simulink model "pha_0_5_servovalve"  (R2023a)
settings: Solver=VariableStepAuto  StartTime=0.0  StopTime=15  RelTol=1e-3
libraries: fl_lib x82, SimscapeFluids_lib x26, nesl_utility x8
(part 1 of 2)
Description:
  | Model contains pump, accumulator, relief valve for pump and accumulator
  | as well as 3-way directional valves. The point of this example is to show how
  | the pressure in accumulator chamber can be controlled to be between 1.4 and 1.5 bars
settings Model: Creator=Dovlica  LastModifiedBy=Dovlica
settings SimscapeCC: SimscapeLogType=all

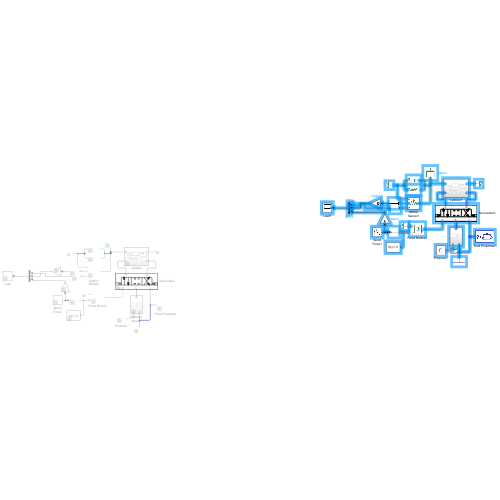
[thumbnail: Simulink's stored preview of the top-level diagram]
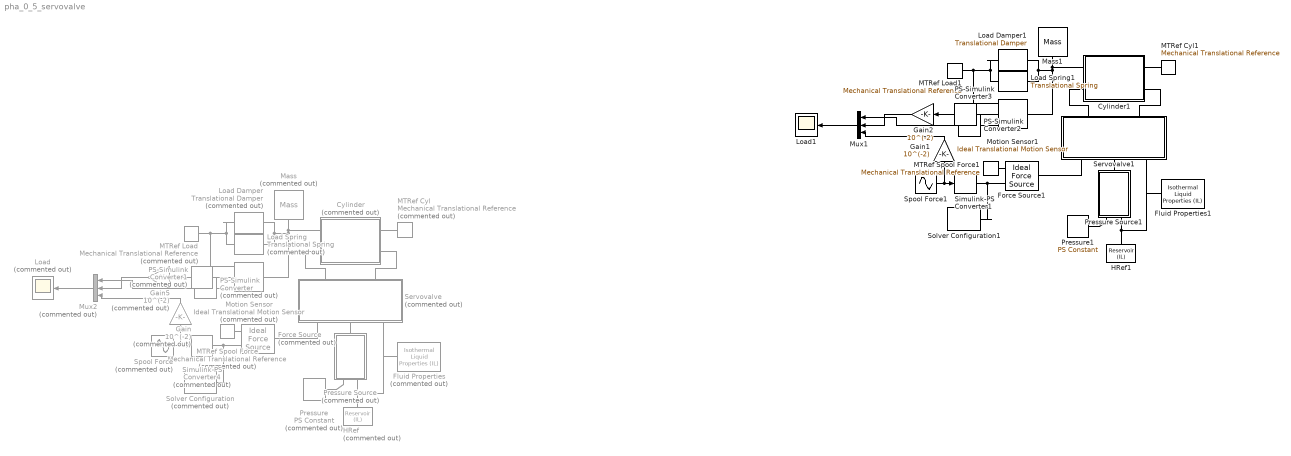
== system pha_0_5_servovalve ==
  " Fluid Properties" : fl_lib/Isothermal Liquid/Utilities/Isothermal Liquid Properties (IL)  Tag=Factory Generic  Commented=on  rho_L_atm=832.816 kg/m^3  bulk_modulus_model=foundation.enum.bulk_modulus_model.const  beta_gain=6  beta_L_atm=1.56078e+09 Pa  nu_atm=(3.9468)*(1) cSt  p_atm=0.101325 MPa  p_min=1 Pa  properties_range_check=simscape.enum.assert.action.error  air_fraction=0.005  polytropic_index=1.0  rho_g_atm=1.225 kg/m^3  air_dissolution_model=simscape.enum.onoff.off  p_crit=3 MPa
      settings: LibrarySourceBlock=fl_lib/Isothermal Liquid/Utilities/Isothermal Liquid Properties (IL)
  " Fluid Properties1" : fl_lib/Isothermal Liquid/Utilities/Isothermal Liquid Properties (IL)  Tag=Factory Generic  rho_L_atm=832.816 kg/m^3  bulk_modulus_model=foundation.enum.bulk_modulus_model.const  beta_gain=6  beta_L_atm=1.56078e+09 Pa  nu_atm=(3.9468)*(1) cSt  p_atm=0.101325 MPa  p_min=1 Pa  properties_range_check=simscape.enum.assert.action.error  air_fraction=0.005  polytropic_index=1.0  rho_g_atm=1.225 kg/m^3  air_dissolution_model=simscape.enum.onoff.off  p_crit=3 MPa
      settings: LibrarySourceBlock=fl_lib/Isothermal Liquid/Utilities/Isothermal Liquid Properties (IL)
  Cylinder : Subsystem  Commented=on
  Cylinder1 : Subsystem
  Force Source : fl_lib/Mechanical/Mechanical Sources/Ideal Force Source  Tag=Factory Generic  Commented=on
  Force Source1 : fl_lib/Mechanical/Mechanical Sources/Ideal Force Source  Tag=Factory Generic
  Gain : Gain  Commented=on  Gain=10^(-2)
  Gain1 : Gain  Gain=10^(-2)
  Gain2 : Gain  Gain=10^(-2)
  Gain5 : Gain  Commented=on  Gain=10^(-2)
  HRef : fl_lib/Isothermal Liquid/Elements/Reservoir (IL)  Tag=Factory Generic  Commented=on  reservoir_type=foundation.enum.constant_controlled.constant  pressure_spec=foundation.enum.pressure_spec.atmospheric  reservoir_pressure=0.101325 MPa
  HRef1 : fl_lib/Isothermal Liquid/Elements/Reservoir (IL)  Tag=Factory Generic  reservoir_type=foundation.enum.constant_controlled.constant  pressure_spec=foundation.enum.pressure_spec.atmospheric  reservoir_pressure=0.101325 MPa
  Load : Scope  Commented=on
  Load Damper : fl_lib/Mechanical/Translational Elements/Translational Damper  Tag=Factory Generic  Commented=on  D=512 N/(m/s)  v_specify=off  v_priority=High  v=0 m/s  v_nominal_specify=off  v_nominal_unit=m/s  v_nominal_value=1  f_specify=off  f_priority=High  f=0 N  f_nominal_specify=off  f_nominal_unit=N  f_nominal_value=1
  Load Damper1 : fl_lib/Mechanical/Translational Elements/Translational Damper  Tag=Factory Generic  D=512 N/(m/s)  v_specify=off  v_priority=High  v=0 m/s  v_nominal_specify=off  v_nominal_unit=m/s  v_nominal_value=1  f_specify=off  f_priority=High  f=0 N  f_nominal_specify=off  f_nominal_unit=N  f_nominal_value=1
  Load Spring : fl_lib/Mechanical/Translational Elements/Translational Spring  Tag=Factory Generic  Commented=on  spr_rate=1.6e5 N/m  v_specify=off  v_priority=High  v=0 m/s  v_nominal_specify=off  v_nominal_unit=m/s  v_nominal_value=1  f_specify=off  f_priority=High  f=0 N  f_nominal_specify=off  f_nominal_unit=N  f_nominal_value=1  x_specify=on  x_priority=High  x=0 m  x_nominal_specify=off  x_nominal_unit=m  x_nominal_value=1
  Load Spring1 : fl_lib/Mechanical/Translational Elements/Translational Spring  Tag=Factory Generic  spr_rate=1.6e5 N/m  v_specify=off  v_priority=High  v=0 m/s  v_nominal_specify=off  v_nominal_unit=m/s  v_nominal_value=1  f_specify=off  f_priority=High  f=0 N  f_nominal_specify=off  f_nominal_unit=N  f_nominal_value=1  x_specify=on  x_priority=High  x=0 m  x_nominal_specify=off  x_nominal_unit=m  x_nominal_value=1
  Load1 : Scope
  MTRef Cyl : fl_lib/Mechanical/Translational Elements/Mechanical Translational Reference  Tag=Factory Generic  Commented=on
  MTRef Cyl1 : fl_lib/Mechanical/Translational Elements/Mechanical Translational Reference  Tag=Factory Generic
  MTRef Load : fl_lib/Mechanical/Translational Elements/Mechanical Translational Reference  Tag=Factory Generic  Commented=on
  MTRef Load1 : fl_lib/Mechanical/Translational Elements/Mechanical Translational Reference  Tag=Factory Generic
  MTRef Spool Force : fl_lib/Mechanical/Translational Elements/Mechanical Translational Reference  Tag=Factory Generic  Commented=on
  MTRef Spool Force1 : fl_lib/Mechanical/Translational Elements/Mechanical Translational Reference  Tag=Factory Generic
  Mass : fl_lib/Mechanical/Translational Elements/Mass  Tag=Factory Generic  Commented=on  mass=25.4 kg  num_ports=foundation.enum.numPorts2.one  v_specify=on  v_priority=High  v=0 m/s  v_nominal_specify=off  v_nominal_unit=m/s  v_nominal_value=1  f_specify=off  f_priority=High  f=0 N  f_nominal_specify=off  f_nominal_unit=N  f_nominal_value=1
  Mass1 : fl_lib/Mechanical/Translational Elements/Mass  Tag=Factory Generic  mass=25.4 kg  num_ports=foundation.enum.numPorts2.one  v_specify=on  v_priority=High  v=0 m/s  v_nominal_specify=off  v_nominal_unit=m/s  v_nominal_value=1  f_specify=off  f_priority=High  f=0 N  f_nominal_specify=off  f_nominal_unit=N  f_nominal_value=1
  Motion Sensor : fl_lib/Mechanical/Mechanical Sensors/Ideal Translational Motion Sensor  Tag=Factory Generic  Commented=on  reference=foundation.enum.MeasurementReference.difference  acceleration_port=false  velocity_port=true  position_port=true  offset=0 m
  Motion Sensor1 : fl_lib/Mechanical/Mechanical Sensors/Ideal Translational Motion Sensor  Tag=Factory Generic  reference=foundation.enum.MeasurementReference.difference  acceleration_port=false  velocity_port=true  position_port=true  offset=0 m
  Mux1 : Mux  Inputs=3
  Mux2 : Mux  Commented=on  Inputs=3
  PS-Simulink Converter : nesl_utility/PS-Simulink Converter  Commented=on  PhysicalDomain=network_engine_domain  SubClassName=ps_output  LeftPortType=input  RightPortType=output  PseudoPeriodic=off  Frequencies=[]  VectorFormat=1-D array  Unit=1  AffineConversion=off
  PS-Simulink Converter1 : nesl_utility/PS-Simulink Converter  Commented=on  PhysicalDomain=network_engine_domain  SubClassName=ps_output  LeftPortType=input  RightPortType=output  PseudoPeriodic=off  Frequencies=[]  VectorFormat=1-D array  Unit=1  AffineConversion=off
  PS-Simulink Converter2 : nesl_utility/PS-Simulink Converter  PhysicalDomain=network_engine_domain  SubClassName=ps_output  LeftPortType=input  RightPortType=output  PseudoPeriodic=off  Frequencies=[]  VectorFormat=1-D array  Unit=1  AffineConversion=off
  PS-Simulink Converter3 : nesl_utility/PS-Simulink Converter  PhysicalDomain=network_engine_domain  SubClassName=ps_output  LeftPortType=input  RightPortType=output  PseudoPeriodic=off  Frequencies=[]  VectorFormat=1-D array  Unit=1  AffineConversion=off
  Pressure : fl_lib/Physical Signals/Sources/PS Constant  Commented=on  constant=75e5
  Pressure Source : Subsystem  Commented=on
  Pressure Source1 : Subsystem
  Pressure1 : fl_lib/Physical Signals/Sources/PS Constant  constant=75e5
  Servovalve : Subsystem  Tag=PublishSubsystem  Commented=on
      mask Display:
      | plot([0;337.311462499201;337.311462499201;0;0], [566.910021007061;566.910021007061;0;0;566.910021007061])
      | %hold on
      | plot([84.6585631370544;241.503668949008], [353;353])
      | plot([84.6585631370544;241.503668949008], [214;214])
      | plot([84.6585631370544;241.503668949008;241.503668949008;84.6585631370544;84.6585631370544], [491;491;76;76;491])
      | plot([84.6585631370544;241.503668949008], [449;449])
      | plot([241.503668949008;210.071657784283], [310;310])
      | plot([210.071657784283;210.071657784283;210.071657784283], [326;295;310.414731502533])
      | plot([241.503668949008;210.071657784283], [257;257])
      | plot([210.071657784283;210.071657784283;210.071657784283], [272;241;236.464468762279])
      | plot([84.6585631370544;115.964594297111], [257;257])
      | plot([115.964594297111;115.964594297111;115.964594297111], [272;241;236.464468762279])
      | plot([84.6585631370544;115.964594297111], [310;310])
      | plot([115.964594297111;115.964594297111;115.964594297111], [326;295;310.414731502533])
      | plot([84.6585631370544;241.503668949008], [185;110])
      | plot([241.503668949008;84.6585631370544], [185;110])
      | plot([84.6585631370544;241.503668949008], [395;395])
      | patch([85.0365031510592;110.547454096377;121.885654516518;85.0365031510592], [110;140;120;110], [0;0;0])
      | plot([85.0365031510592;110.547454096377;121.885654516518;85.0365031510592], [110;140;120;110])
      | patch([240.936758928001;204.087607562542;215.425807982683;240.936758928001], [109;120;140;109], [0;0;0])
      | plot([240.936758928001;204.087607562542;215.425807982683;240.936758928001], [109;120;140;109])
      | patch([83.6507230997086;127.554754726589;127.554754726589;83.6507230997086], [451;461;440;451], [0;0;0])
      | plot([83.6507230997086;127.554754726589;127.554754726589;83.6507230997086], [451;461;440;451])
      | patch([245.283069089055;201.253057457507;201.253057457507;245.283069089055], [394;405;384;394], [0;0;0])
      | plot([245.283069089055;201.253057457507;201.253057457507;245.283069089055], [394;405;384;394])
      | 
      | plot([241.5; 241.5;201; 201], [491; 566; 566; 491])
      | patch([241; 205; 222; 241], [525;525;495;525], [0;0;0]')
      | plot([241.5; 241.5;201; 201], [76; 0; 0; 76])
      | patch([241; 205; 222; 241], [40;40;70;40], [0;0;0])
      | %plot([241.5; 201], [11; 26])
      | %plot([241.5; 201], [561; 541])
      | 
      | %plot([127; 85;127; 85], [491; 511; 531; 551])
      | %plot([127; 85;127; 85], [76; 56; 36; 16])
      | %hold off
      | 
      | 
      | color('red');
      | port_label('LConn', 1,'A')
      | port_label('LConn', 2,'B')
      | port_label('RConn', 1,'S')
      | port_label('RConn', 2,'P')
      | port_label('RConn', 3,'T')
  Servovalve1 : Subsystem  Tag=PublishSubsystem
      mask Display:
      | plot([0;337.311462499201;337.311462499201;0;0], [566.910021007061;566.910021007061;0;0;566.910021007061])
      | %hold on
      | plot([84.6585631370544;241.503668949008], [353;353])
      | plot([84.6585631370544;241.503668949008], [214;214])
      | plot([84.6585631370544;241.503668949008;241.503668949008;84.6585631370544;84.6585631370544], [491;491;76;76;491])
      | plot([84.6585631370544;241.503668949008], [449;449])
      | plot([241.503668949008;210.071657784283], [310;310])
      | plot([210.071657784283;210.071657784283;210.071657784283], [326;295;310.414731502533])
      | plot([241.503668949008;210.071657784283], [257;257])
      | plot([210.071657784283;210.071657784283;210.071657784283], [272;241;236.464468762279])
      | plot([84.6585631370544;115.964594297111], [257;257])
      | plot([115.964594297111;115.964594297111;115.964594297111], [272;241;236.464468762279])
      | plot([84.6585631370544;115.964594297111], [310;310])
      | plot([115.964594297111;115.964594297111;115.964594297111], [326;295;310.414731502533])
      | plot([84.6585631370544;241.503668949008], [185;110])
      | plot([241.503668949008;84.6585631370544], [185;110])
      | plot([84.6585631370544;241.503668949008], [395;395])
      | patch([85.0365031510592;110.547454096377;121.885654516518;85.0365031510592], [110;140;120;110], [0;0;0])
      | plot([85.0365031510592;110.547454096377;121.885654516518;85.0365031510592], [110;140;120;110])
      | patch([240.936758928001;204.087607562542;215.425807982683;240.936758928001], [109;120;140;109], [0;0;0])
      | plot([240.936758928001;204.087607562542;215.425807982683;240.936758928001], [109;120;140;109])
      | patch([83.6507230997086;127.554754726589;127.554754726589;83.6507230997086], [451;461;440;451], [0;0;0])
      | plot([83.6507230997086;127.554754726589;127.554754726589;83.6507230997086], [451;461;440;451])
      | patch([245.283069089055;201.253057457507;201.253057457507;245.283069089055], [394;405;384;394], [0;0;0])
      | plot([245.283069089055;201.253057457507;201.253057457507;245.283069089055], [394;405;384;394])
      | 
      | plot([241.5; 241.5;201; 201], [491; 566; 566; 491])
      | patch([241; 205; 222; 241], [525;525;495;525], [0;0;0]')
      | plot([241.5; 241.5;201; 201], [76; 0; 0; 76])
      | patch([241; 205; 222; 241], [40;40;70;40], [0;0;0])
      | %plot([241.5; 201], [11; 26])
      | %plot([241.5; 201], [561; 541])
      | 
      | %plot([127; 85;127; 85], [491; 511; 531; 551])
      | %plot([127; 85;127; 85], [76; 56; 36; 16])
      | %hold off
      | 
      | 
      | color('red');
      | port_label('LConn', 1,'A')
      | port_label('LConn', 2,'B')
      | port_label('RConn', 1,'S')
      | port_label('RConn', 2,'P')
      | port_label('RConn', 3,'T')
  Simulink-PS Converter1 : nesl_utility/Simulink-PS Converter  PhysicalDomain=network_engine_domain  SubClassName=ps_input  LeftPortType=input  RightPortType=output  PseudoPeriodic=off  Frequencies=[]  NoiseDistribution=none  NoiseParameters=[]  Unit=1  AffineConversion=off  FilteringAndDerivatives=zero  SimscapeFilterOrder=1  InputFilterTimeConstant=.001  UdotUserProvided=0
  Simulink-PS Converter4 : nesl_utility/Simulink-PS Converter  Commented=on  PhysicalDomain=network_engine_domain  SubClassName=ps_input  LeftPortType=input  RightPortType=output  PseudoPeriodic=off  Frequencies=[]  NoiseDistribution=none  NoiseParameters=[]  Unit=1  AffineConversion=off  FilteringAndDerivatives=zero  SimscapeFilterOrder=1  InputFilterTimeConstant=.001  UdotUserProvided=0
  Solver Configuration : nesl_utility/Solver Configuration  Commented=on  PhysicalDomain=network_engine_domain  SubClassName=solver  LeftPortType=input  RightPortType=generic  Tones=[]  Harmonics=[]  SimulateNoise=off  Profile=off  UseLocalSampling=off  EnableSwitchedLinearOptims=on  FrequencyDomain=off  UseCCode=off  RelTol=0.001  AbsTol=1e-06  MinStep=1e-09  ToWorkspace=off  RevertToSquareIcSolve=off  NumHomotopyIterations=100  PhasorMode=off  PhasorModeNumHarmonics=1  ConsistencySolver=NEWTON_XTOL_AFTER_FTOL  IndexReductionMethod=DerivativeReplacement  DoDC=off  ResidualTolerance=1e-9  ConsistencyTolSource=GLOBAL  ConsistencyAbsTol=0.001  ConsistencyRelTol=0.001  ConsistencyTolFactor=0.001  UseLocalSolver=off  LocalSolverChoice=NE_BACKWARD_EULER_ADVANCER  ResolveIndetEquations=on  FunctionEvalNumThread=1  LocalSolverSampleTime=.001  DoFixedCost=off  MaxNonlinIter=3  MaxModeIter=2  ComputeImpulses=off  ImpulseIterations=2  LinearAlgebra=auto  LinearAlgebraNumThread=0  EquationFormulation=NE_TIME_EF  DelaysMemoryBudget=1024  AutomaticFiltering=on  FilteringTimeConstant=0.001  PartitionStorageMethod=AS_NEEDED  PartitionMemoryBudget=1024  PartitionMethod=FAST
  Solver Configuration1 : nesl_utility/Solver Configuration  PhysicalDomain=network_engine_domain  SubClassName=solver  LeftPortType=input  RightPortType=generic  Tones=[]  Harmonics=[]  SimulateNoise=off  Profile=off  UseLocalSampling=off  EnableSwitchedLinearOptims=on  FrequencyDomain=off  UseCCode=off  RelTol=0.001  AbsTol=1e-06  MinStep=1e-09  ToWorkspace=off  RevertToSquareIcSolve=off  NumHomotopyIterations=100  PhasorMode=off  PhasorModeNumHarmonics=1  ConsistencySolver=NEWTON_XTOL_AFTER_FTOL  IndexReductionMethod=DerivativeReplacement  DoDC=off  ResidualTolerance=1e-9  ConsistencyTolSource=GLOBAL  ConsistencyAbsTol=0.001  ConsistencyRelTol=0.001  ConsistencyTolFactor=0.001  UseLocalSolver=off  LocalSolverChoice=NE_BACKWARD_EULER_ADVANCER  ResolveIndetEquations=on  FunctionEvalNumThread=1  LocalSolverSampleTime=.001  DoFixedCost=off  MaxNonlinIter=3  MaxModeIter=2  ComputeImpulses=off  ImpulseIterations=2  LinearAlgebra=auto  LinearAlgebraNumThread=0  EquationFormulation=NE_TIME_EF  DelaysMemoryBudget=1024  AutomaticFiltering=on  FilteringTimeConstant=0.001  PartitionStorageMethod=AS_NEEDED  PartitionMemoryBudget=1024  PartitionMethod=FAST
  Spool Force : Sin  Commented=on  Amplitude=12  Frequency=10  SampleTime=0
  Spool Force1 : Sin  Amplitude=12  Frequency=10  SampleTime=0
  wires:
  PS-Simulink Converter/1 -> Mux2/1
  Gain5/1 -> Mux2/2
  Gain/1 -> Mux2/3
  Spool Force/1 -> Gain/1, Simulink-PS Converter4/1
  Mux2/1 -> Load/1
  PS-Simulink Converter1/1 -> Gain5/1
  PS-Simulink Converter2/1 -> Mux1/1
  Gain2/1 -> Mux1/2
  Gain1/1 -> Mux1/3
  Spool Force1/1 -> Gain1/1, Simulink-PS Converter1/1
  Mux1/1 -> Load1/1
  PS-Simulink Converter3/1 -> Gain2/1
  connections:
  HRef/LConn1 -- " Fluid Properties"/RConn1 -- Servovalve/RConn3 -- Pressure Source/RConn2
  Solver Configuration/RConn1 -- Force Source/RConn1 -- Simulink-PS Converter4/RConn1
  MTRef Load/LConn1 -- Load Damper/RConn1 -- Load Spring/RConn1 -- Motion Sensor/RConn1
  Load Spring/LConn1 -- Mass/LConn1 -- Cylinder/RConn1 -- Motion Sensor/LConn1 -- Load Damper/LConn1
  MTRef Cyl/LConn1 -- Cylinder/LConn1
  Pressure/RConn1 -- Pressure Source/RConn1
  Servovalve/LConn1 -- Cylinder/RConn2
  PS-Simulink Converter1/LConn1 -- Motion Sensor/RConn2
  Servovalve/RConn1 -- Force Source/LConn1
  Motion Sensor/RConn3 -- PS-Simulink Converter/LConn1
  Servovalve/RConn2 -- Pressure Source/LConn1
  Servovalve/LConn2 -- Cylinder/LConn2
  MTRef Spool Force/LConn1 -- Force Source/RConn2
  HRef1/LConn1 -- " Fluid Properties1"/RConn1 -- Servovalve1/RConn3 -- Pressure Source1/RConn2
  Solver Configuration1/RConn1 -- Force Source1/RConn1 -- Simulink-PS Converter1/RConn1
  MTRef Load1/LConn1 -- Load Damper1/RConn1 -- Load Spring1/RConn1 -- Motion Sensor1/RConn1
  Load Spring1/LConn1 -- Mass1/LConn1 -- Cylinder1/RConn1 -- Motion Sensor1/LConn1 -- Load Damper1/LConn1
  MTRef Cyl1/LConn1 -- Cylinder1/LConn1
  Pressure1/RConn1 -- Pressure Source1/RConn1
  Servovalve1/LConn1 -- Cylinder1/RConn2
  PS-Simulink Converter3/LConn1 -- Motion Sensor1/RConn2
  Servovalve1/RConn1 -- Force Source1/LConn1
  Motion Sensor1/RConn3 -- PS-Simulink Converter2/LConn1
  Servovalve1/RConn2 -- Pressure Source1/LConn1
  Servovalve1/LConn2 -- Cylinder1/LConn2
  MTRef Spool Force1/LConn1 -- Force Source1/RConn2

== system pha_0_5_servovalve/Cylinder ==
  Cylinder : SimscapeFluids_lib/Isothermal Liquid/Actuators/Double-Acting Actuator (IL)  Tag=Factory Generic  mech_orientation=-1  piston_area_A=20 cm^2  piston_area_B=20 cm^2  stroke=0.3 m  dead_volume_A=1e-4 m^3  dead_volume_B=1e-4 m^3  pressure_spec=foundation.enum.pressure_spec.atmospheric  environment_pressure=0.101325 MPa  hardstop_model=3  stiff_coeff=1e6 N/m  damping_coeff=210 N/(m/s)  transition=0.1 mm  coeff_rest=0.7  v_tol=0.001 m/s  f_tol=0.001 N  cushion_A_spec=false  area_plunger_A=1e-4 m^2  length_plunger_A=1e-3 m  area_cushion_orifice_A=1e-6 m^2  area_leak_plunger_A=1e-7 m^2  p_crack_differential_A=0.01 MPa  press_max_differential_A=0.1 MPa  check_valve_area_max_A=1e-4 m^2  check_valve_area_leak_A=1e-10 m^2  smoothing_factor_A=0  cushion_B_spec=false  area_plunger_B=1e-4 m^2  length_plunger_B=1e-3 m  area_cushion_orifice_B=1e-6 m^2  area_leak_plunger_B=1e-7 m^2  p_crack_differential_B=0.01 MPa  press_max_differential_B=0.1 MPa  check_valve_area_max_B=1e-4 m^2  check_valve_area_leak_B=1e-10 m^2  smoothing_factor_B=0  friction_spec=false  breakaway_Coulomb_ratio=1.2  breakaway_velocity=0.1 m/s  preload_force=20 N  Coulomb_coeff=1e-6 N/Pa  viscous_coeff=100 N*s/m  leakage_spec=false  clearance=1e-4 m  piston_length=0.01 m  displacement_spec=foundation.enum.DisplacementSpec.Calculate  x0=-(0.15) m  dynamic_compressibility=true  p0_A=0 + 101325 Pa  p0_B=0 + 101325 Pa
      settings: LibrarySourceBlock=SimscapeFluids_lib/Isothermal Liquid/Actuators/Double-Acting Actuator (IL)  InternalSimscapePortConfiguration="{\"Bottom\":[],\"Left\":[{\"id\":\"C\",\"label\":\"C\",\"type\":\"foundation.mechanical.translational.translational\"},{\"id\":\"A\",\"label\":\"A\",\"type\":\"foundation.isothermal_liquid.isothermal_liquid\"}],\"Right\":[{\"id\":\"p_out\",\"label\":\"p\",\"type\":\"output\"},{\"id\":\"R\",\"label\":\"R\",\"type\":\"foundation.mechanical.translational.translational\"},{\"id\":\"B\",\"label\":\"B\",\"type\":\"foundation.isothermal_liquid.isothermal_liquid\"}],\"Top\":[]}"
  R : PMIOPort  Side=Right
  C : PMIOPort  Port=2  Side=Left
  B : PMIOPort  Port=3  Side=Right
  A : PMIOPort  Port=4  Side=Left
  connections:
  C/RConn1 -- Cylinder/LConn1
  A/RConn1 -- Cylinder/LConn2
  R/RConn1 -- Cylinder/RConn2
  B/RConn1 -- Cylinder/RConn3

== system pha_0_5_servovalve/Cylinder1 ==
  Cylinder : SimscapeFluids_lib/Isothermal Liquid/Actuators/Double-Acting Actuator (IL)  Tag=Factory Generic  mech_orientation=-1  piston_area_A=20 cm^2  piston_area_B=20 cm^2  stroke=0.3 m  dead_volume_A=1e-4 m^3  dead_volume_B=1e-4 m^3  pressure_spec=foundation.enum.pressure_spec.atmospheric  environment_pressure=0.101325 MPa  hardstop_model=3  stiff_coeff=1e6 N/m  damping_coeff=210 N/(m/s)  transition=0.1 mm  coeff_rest=0.7  v_tol=0.001 m/s  f_tol=0.001 N  cushion_A_spec=false  area_plunger_A=1e-4 m^2  length_plunger_A=1e-3 m  area_cushion_orifice_A=1e-6 m^2  area_leak_plunger_A=1e-7 m^2  p_crack_differential_A=0.01 MPa  press_max_differential_A=0.1 MPa  check_valve_area_max_A=1e-4 m^2  check_valve_area_leak_A=1e-10 m^2  smoothing_factor_A=0  cushion_B_spec=false  area_plunger_B=1e-4 m^2  length_plunger_B=1e-3 m  area_cushion_orifice_B=1e-6 m^2  area_leak_plunger_B=1e-7 m^2  p_crack_differential_B=0.01 MPa  press_max_differential_B=0.1 MPa  check_valve_area_max_B=1e-4 m^2  check_valve_area_leak_B=1e-10 m^2  smoothing_factor_B=0  friction_spec=false  breakaway_Coulomb_ratio=1.2  breakaway_velocity=0.1 m/s  preload_force=20 N  Coulomb_coeff=1e-6 N/Pa  viscous_coeff=100 N*s/m  leakage_spec=false  clearance=1e-4 m  piston_length=0.01 m  displacement_spec=foundation.enum.DisplacementSpec.Calculate  x0=-(0.15) m  dynamic_compressibility=true  p0_A=0 + 101325 Pa  p0_B=0 + 101325 Pa
      settings: LibrarySourceBlock=SimscapeFluids_lib/Isothermal Liquid/Actuators/Double-Acting Actuator (IL)  InternalSimscapePortConfiguration="{\"Bottom\":[],\"Left\":[{\"id\":\"C\",\"label\":\"C\",\"type\":\"foundation.mechanical.translational.translational\"},{\"id\":\"A\",\"label\":\"A\",\"type\":\"foundation.isothermal_liquid.isothermal_liquid\"}],\"Right\":[{\"id\":\"p_out\",\"label\":\"p\",\"type\":\"output\"},{\"id\":\"R\",\"label\":\"R\",\"type\":\"foundation.mechanical.translational.translational\"},{\"id\":\"B\",\"label\":\"B\",\"type\":\"foundation.isothermal_liquid.isothermal_liquid\"}],\"Top\":[]}"
  R : PMIOPort  Side=Right
  C : PMIOPort  Port=2  Side=Left
  B : PMIOPort  Port=3  Side=Right
  A : PMIOPort  Port=4  Side=Left
  connections:
  C/RConn1 -- Cylinder/LConn1
  A/RConn1 -- Cylinder/LConn2
  R/RConn1 -- Cylinder/RConn2
  B/RConn1 -- Cylinder/RConn3

== system pha_0_5_servovalve/Pressure Source ==
  Pressure Source : fl_lib/Isothermal Liquid/Sources/Pressure Source (IL)  Tag=Factory Generic  source_type=foundation.enum.constant_controlled.controlled  pressure_differential=0 MPa
      settings: InternalSimscapePortConfiguration="{\"Bottom\":[],\"Left\":[{\"id\":\"A\",\"label\":\"A\",\"type\":\"foundation.isothermal_liquid.isothermal_liquid\"},{\"id\":\"P\",\"label\":\"P\",\"type\":\"input\"}],\"Right\":[{\"id\":\"B\",\"label\":\"B\",\"type\":\"foundation.isothermal_liquid.isothermal_liquid\"}],\"Top\":[]}"
  B : PMIOPort  Side=Left
  P : PMIOPort  Port=2  Side=Right
  A : PMIOPort  Port=3  Side=Right
  connections:
  P/RConn1 -- Pressure Source/LConn2
  B/RConn1 -- Pressure Source/RConn1
  Pressure Source/LConn1 -- A/RConn1

== system pha_0_5_servovalve/Pressure Source1 ==
  Pressure Source : fl_lib/Isothermal Liquid/Sources/Pressure Source (IL)  Tag=Factory Generic  source_type=foundation.enum.constant_controlled.controlled  pressure_differential=0 MPa
      settings: InternalSimscapePortConfiguration="{\"Bottom\":[],\"Left\":[{\"id\":\"A\",\"label\":\"A\",\"type\":\"foundation.isothermal_liquid.isothermal_liquid\"},{\"id\":\"P\",\"label\":\"P\",\"type\":\"input\"}],\"Right\":[{\"id\":\"B\",\"label\":\"B\",\"type\":\"foundation.isothermal_liquid.isothermal_liquid\"}],\"Top\":[]}"
  B : PMIOPort  Side=Left
  P : PMIOPort  Port=2  Side=Right
  A : PMIOPort  Port=3  Side=Right
  connections:
  P/RConn1 -- Pressure Source/LConn2
  B/RConn1 -- Pressure Source/RConn1
  Pressure Source/LConn1 -- A/RConn1

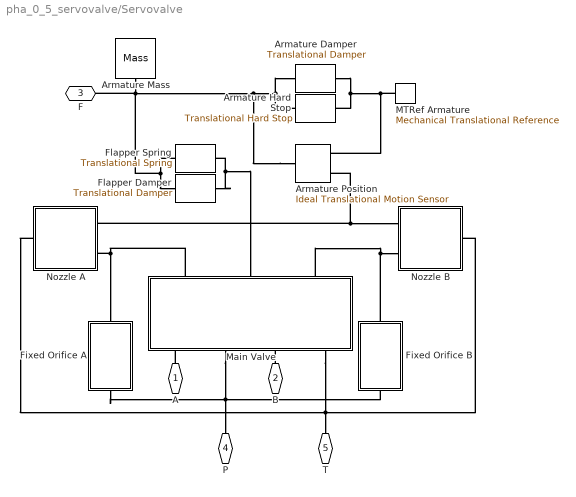
== system pha_0_5_servovalve/Servovalve ==
  Armature Mass : fl_lib/Mechanical/Translational Elements/Mass  Tag=Factory Generic  mass=0.035 kg  num_ports=foundation.enum.numPorts2.one  v_specify=on  v_priority=High  v=0 m/s  v_nominal_specify=off  v_nominal_unit=m/s  v_nominal_value=1  f_specify=off  f_priority=High  f=0 N  f_nominal_specify=off  f_nominal_unit=N  f_nominal_value=1
  Armature Position : fl_lib/Mechanical/Mechanical Sensors/Ideal Translational Motion Sensor  Tag=Factory Generic  reference=foundation.enum.MeasurementReference.difference  acceleration_port=false  velocity_port=true  position_port=true  offset=0 m
  Armature Damper : fl_lib/Mechanical/Translational Elements/Translational Damper  Tag=Factory Generic  D=12.5 N/(m/s)  v_specify=off  v_priority=High  v=0 m/s  v_nominal_specify=off  v_nominal_unit=m/s  v_nominal_value=1  f_specify=off  f_priority=High  f=0 N  f_nominal_specify=off  f_nominal_unit=N  f_nominal_value=1
  Armature Hard Stop : fl_lib/Mechanical/Translational Elements/Translational Hard Stop  Tag=Factory Generic  upper_bnd=0.5 mm  lower_bnd=-0.5 mm  model=3  stiff_up=1e+06 N/m  stiff_low=1e+06 N/m  D_up=150 N/(m/s)  D_low=150 N/(m/s)  transition=0.1 mm  coeff_rest=0.7  v_tol=0.001 m/s  f_tol=0.001 N  x_specify=on  x_priority=High  x=0 m  x_nominal_specify=off  x_nominal_unit=m  x_nominal_value=1  v_specify=off  v_priority=High  v=0 m/s  v_nominal_specify=off  v_nominal_unit=m/s  v_nominal_value=1  f_specify=off  f_priority=High  f=0 N  f_nominal_specify=off  f_nominal_unit=N  f_nominal_value=1  M_specify=off  M_priority=None  M=0
  Fixed Orifice A : Subsystem
  Fixed Orifice B : Subsystem
  Flapper Damper : fl_lib/Mechanical/Translational Elements/Translational Damper  Tag=Factory Generic  D=51 N/(m/s)  v_specify=off  v_priority=High  v=0 m/s  v_nominal_specify=off  v_nominal_unit=m/s  v_nominal_value=1  f_specify=off  f_priority=High  f=0 N  f_nominal_specify=off  f_nominal_unit=N  f_nominal_value=1
  Flapper Spring : fl_lib/Mechanical/Translational Elements/Translational Spring  Tag=Factory Generic  spr_rate=1200 N/m  v_specify=off  v_priority=High  v=0 m/s  v_nominal_specify=off  v_nominal_unit=m/s  v_nominal_value=1  f_specify=off  f_priority=High  f=0 N  f_nominal_specify=off  f_nominal_unit=N  f_nominal_value=1  x_specify=on  x_priority=High  x=0 m  x_nominal_specify=off  x_nominal_unit=m  x_nominal_value=1
  MTRef Armature : fl_lib/Mechanical/Translational Elements/Mechanical Translational Reference  Tag=Factory Generic
  Main Valve : Subsystem  Tag=PublishSubsystem
  Nozzle A : Subsystem
  Nozzle B : Subsystem
  A : PMIOPort  Side=Left
  B : PMIOPort  Port=2  Side=Left
  F : PMIOPort  Port=3  Side=Right
  P : PMIOPort  Port=4  Side=Right
  T : PMIOPort  Port=5  Side=Right
  connections:
  Main Valve/RConn2 -- Fixed Orifice B/LConn1 -- Fixed Orifice A/LConn1 -- P/RConn1
  Armature Position/LConn1 -- Flapper Spring/LConn1 -- Flapper Damper/LConn1 -- F/RConn1 -- Armature Mass/LConn1 -- Armature Damper/LConn1 -- Armature Hard Stop/LConn1
  A/RConn1 -- Main Valve/RConn1
  B/RConn1 -- Main Valve/RConn3
  Flapper Damper/RConn1 -- Flapper Spring/RConn1 -- Main Valve/LConn2
  MTRef Armature/LConn1 -- Armature Position/RConn1 -- Armature Damper/RConn1 -- Armature Hard Stop/RConn1
  Main Valve/LConn1 -- Nozzle A/LConn2 -- Fixed Orifice A/RConn1
  Armature Position/RConn3 -- Nozzle B/LConn1 -- Nozzle A/LConn1
  Fixed Orifice B/RConn1 -- Main Valve/LConn3 -- Nozzle B/LConn2
  Nozzle A/RConn1 -- Nozzle B/RConn1 -- T/RConn1 -- Main Valve/RConn4

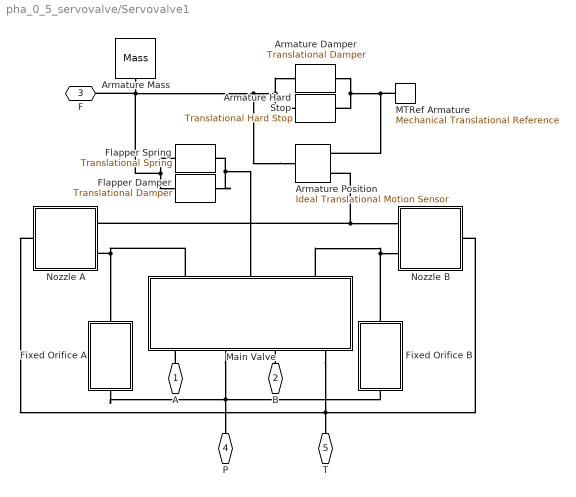
== system pha_0_5_servovalve/Servovalve1 ==
  Armature Mass : fl_lib/Mechanical/Translational Elements/Mass  Tag=Factory Generic  mass=0.035 kg  num_ports=foundation.enum.numPorts2.one  v_specify=on  v_priority=High  v=0 m/s  v_nominal_specify=off  v_nominal_unit=m/s  v_nominal_value=1  f_specify=off  f_priority=High  f=0 N  f_nominal_specify=off  f_nominal_unit=N  f_nominal_value=1
  Armature Position : fl_lib/Mechanical/Mechanical Sensors/Ideal Translational Motion Sensor  Tag=Factory Generic  reference=foundation.enum.MeasurementReference.difference  acceleration_port=false  velocity_port=true  position_port=true  offset=0 m
  Armature Damper : fl_lib/Mechanical/Translational Elements/Translational Damper  Tag=Factory Generic  D=12.5 N/(m/s)  v_specify=off  v_priority=High  v=0 m/s  v_nominal_specify=off  v_nominal_unit=m/s  v_nominal_value=1  f_specify=off  f_priority=High  f=0 N  f_nominal_specify=off  f_nominal_unit=N  f_nominal_value=1
  Armature Hard Stop : fl_lib/Mechanical/Translational Elements/Translational Hard Stop  Tag=Factory Generic  upper_bnd=0.5 mm  lower_bnd=-0.5 mm  model=3  stiff_up=1e+06 N/m  stiff_low=1e+06 N/m  D_up=150 N/(m/s)  D_low=150 N/(m/s)  transition=0.1 mm  coeff_rest=0.7  v_tol=0.001 m/s  f_tol=0.001 N  x_specify=on  x_priority=High  x=0 m  x_nominal_specify=off  x_nominal_unit=m  x_nominal_value=1  v_specify=off  v_priority=High  v=0 m/s  v_nominal_specify=off  v_nominal_unit=m/s  v_nominal_value=1  f_specify=off  f_priority=High  f=0 N  f_nominal_specify=off  f_nominal_unit=N  f_nominal_value=1  M_specify=off  M_priority=None  M=0
  Fixed Orifice A : Subsystem
  Fixed Orifice B : Subsystem
  Flapper Damper : fl_lib/Mechanical/Translational Elements/Translational Damper  Tag=Factory Generic  D=51 N/(m/s)  v_specify=off  v_priority=High  v=0 m/s  v_nominal_specify=off  v_nominal_unit=m/s  v_nominal_value=1  f_specify=off  f_priority=High  f=0 N  f_nominal_specify=off  f_nominal_unit=N  f_nominal_value=1
  Flapper Spring : fl_lib/Mechanical/Translational Elements/Translational Spring  Tag=Factory Generic  spr_rate=1200 N/m  v_specify=off  v_priority=High  v=0 m/s  v_nominal_specify=off  v_nominal_unit=m/s  v_nominal_value=1  f_specify=off  f_priority=High  f=0 N  f_nominal_specify=off  f_nominal_unit=N  f_nominal_value=1  x_specify=on  x_priority=High  x=0 m  x_nominal_specify=off  x_nominal_unit=m  x_nominal_value=1
  MTRef Armature : fl_lib/Mechanical/Translational Elements/Mechanical Translational Reference  Tag=Factory Generic
  Main Valve : Subsystem  Tag=PublishSubsystem
  Nozzle A : Subsystem
  Nozzle B : Subsystem
  A : PMIOPort  Side=Left
  B : PMIOPort  Port=2  Side=Left
  F : PMIOPort  Port=3  Side=Right
  P : PMIOPort  Port=4  Side=Right
  T : PMIOPort  Port=5  Side=Right
  connections:
  Main Valve/RConn2 -- Fixed Orifice B/LConn1 -- Fixed Orifice A/LConn1 -- P/RConn1
  Armature Position/LConn1 -- Flapper Spring/LConn1 -- Flapper Damper/LConn1 -- F/RConn1 -- Armature Mass/LConn1 -- Armature Damper/LConn1 -- Armature Hard Stop/LConn1
  A/RConn1 -- Main Valve/RConn1
  B/RConn1 -- Main Valve/RConn3
  Flapper Damper/RConn1 -- Flapper Spring/RConn1 -- Main Valve/LConn2
  MTRef Armature/LConn1 -- Armature Position/RConn1 -- Armature Damper/RConn1 -- Armature Hard Stop/RConn1
  Main Valve/LConn1 -- Nozzle A/LConn2 -- Fixed Orifice A/RConn1
  Armature Position/RConn3 -- Nozzle B/LConn1 -- Nozzle A/LConn1
  Fixed Orifice B/RConn1 -- Main Valve/LConn3 -- Nozzle B/LConn2
  Nozzle A/RConn1 -- Nozzle B/RConn1 -- T/RConn1 -- Main Valve/RConn4

== system pha_0_5_servovalve/Servovalve/Fixed Orifice A ==
  Fixed Orifice A : SimscapeFluids_lib/Isothermal Liquid/Valves & Orifices/Orifices/Orifice (IL)  Tag=Factory Generic  orifice_type=1  constant_orifice_spec=fluids.isothermal_liquid.valves_orifices.orifices.enum.constant_orifice_spec.area  variable_orifice_spec=fluids.isothermal_liquid.valves_orifices.orifices.enum.orifice_spec.linear  orifice_area_constant=2 mm^2  p_diff_TLU_constant=[-4, -3, -2, -1, -.5, 0, .5, 1, 2, 3, 4] MPa  vol_flow_TLU_constant=[-2.44, -2.12, -1.68, -1.22, -.84, 0, .85, 1.21, 1.7, 2.09, 2.41] .* 1e-3 m^3/s  S_min=0 m  del_S=5e-3 m  open_orientation=fluids.isothermal_liquid.valves_orifices.orifices.enum.orifice_orientation.positive  area_max=1e-4 m^2  area_leak=1e-10 m^2  S_TLU=[0, .002, .004, .007, .017] m  orifice_area_TLU=[1e-09, 2.0352e-07, 4.0736e-05, .00011438, .00034356] m^2  area=inf mm^2  Cd=0.7  Re_c=150  smoothing_factor=0.01  pressure_recovery=false  S_vol_flow_TLU=[0, .002, .004, .007, .017] m  p_diff_TLU=[.3, .5, .7] MPa  vol_flow_TLU=1e-3 * [1.7e-05, 2e-05, 2.6e-05; .0035, .0045, .0053; .7, .9, 1.06; 1.96, 2.5, 3; 6, 7.7, 9.13] m^3/s  enable_faults=simscape.enum.onoff.off  fault_action=fluids.enum.FaultOpening.Closed  external_fault=fluids.enum.FaultExternalTrigger.Off  temporal_fault=simscape.enum.onoff.off  fault_time=5 s  report_fault=simscape.enum.assert.action.none
      settings: InternalSimscapePortConfiguration="{\"Bottom\":[],\"Left\":[{\"id\":\"A\",\"label\":\"A\",\"type\":\"foundation.isothermal_liquid.isothermal_liquid\"}],\"Right\":[{\"id\":\"B\",\"label\":\"B\",\"type\":\"foundation.isothermal_liquid.isothermal_liquid\"}],\"Top\":[]}"
  B : PMIOPort  Side=Right
  A : PMIOPort  Port=2  Side=Left
  connections:
  A/RConn1 -- Fixed Orifice A/LConn1
  B/RConn1 -- Fixed Orifice A/RConn1

== system pha_0_5_servovalve/Servovalve/Fixed Orifice B ==
  Fixed Orifice B : SimscapeFluids_lib/Isothermal Liquid/Valves & Orifices/Orifices/Orifice (IL)  Tag=Factory Generic  orifice_type=1  constant_orifice_spec=fluids.isothermal_liquid.valves_orifices.orifices.enum.constant_orifice_spec.area  variable_orifice_spec=fluids.isothermal_liquid.valves_orifices.orifices.enum.orifice_spec.linear  orifice_area_constant=2 mm^2  p_diff_TLU_constant=[-4, -3, -2, -1, -.5, 0, .5, 1, 2, 3, 4] MPa  vol_flow_TLU_constant=[-2.44, -2.12, -1.68, -1.22, -.84, 0, .85, 1.21, 1.7, 2.09, 2.41] .* 1e-3 m^3/s  S_min=0 m  del_S=5e-3 m  open_orientation=fluids.isothermal_liquid.valves_orifices.orifices.enum.orifice_orientation.positive  area_max=1e-4 m^2  area_leak=1e-10 m^2  S_TLU=[0, .002, .004, .007, .017] m  orifice_area_TLU=[1e-09, 2.0352e-07, 4.0736e-05, .00011438, .00034356] m^2  area=inf mm^2  Cd=0.7  Re_c=150  smoothing_factor=0.01  pressure_recovery=false  S_vol_flow_TLU=[0, .002, .004, .007, .017] m  p_diff_TLU=[.3, .5, .7] MPa  vol_flow_TLU=1e-3 * [1.7e-05, 2e-05, 2.6e-05; .0035, .0045, .0053; .7, .9, 1.06; 1.96, 2.5, 3; 6, 7.7, 9.13] m^3/s  enable_faults=simscape.enum.onoff.off  fault_action=fluids.enum.FaultOpening.Closed  external_fault=fluids.enum.FaultExternalTrigger.Off  temporal_fault=simscape.enum.onoff.off  fault_time=5 s  report_fault=simscape.enum.assert.action.none
      settings: InternalSimscapePortConfiguration="{\"Bottom\":[],\"Left\":[{\"id\":\"A\",\"label\":\"A\",\"type\":\"foundation.isothermal_liquid.isothermal_liquid\"}],\"Right\":[{\"id\":\"B\",\"label\":\"B\",\"type\":\"foundation.isothermal_liquid.isothermal_liquid\"}],\"Top\":[]}"
  B : PMIOPort  Side=Right
  A : PMIOPort  Port=2  Side=Left
  connections:
  A/RConn1 -- Fixed Orifice B/LConn1
  B/RConn1 -- Fixed Orifice B/RConn1

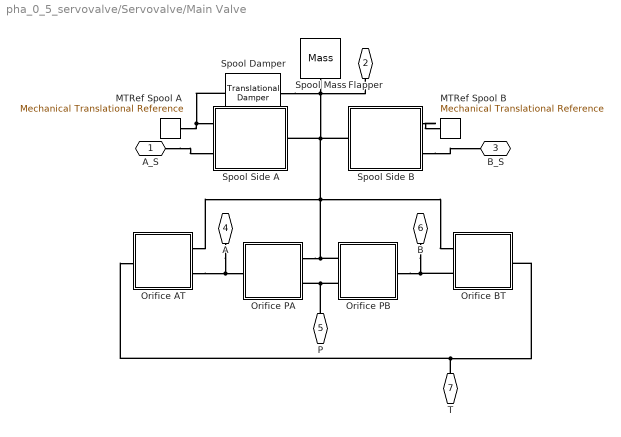
== system pha_0_5_servovalve/Servovalve/Main Valve ==
  MTRef Spool A : fl_lib/Mechanical/Translational Elements/Mechanical Translational Reference  Tag=Factory Generic
  MTRef Spool B : fl_lib/Mechanical/Translational Elements/Mechanical Translational Reference  Tag=Factory Generic
  Orifice AT : Subsystem  Tag=PublishSubsystem
  Orifice BT : Subsystem
  Orifice PA : Subsystem
  Orifice PB : Subsystem
  Spool Damper : fl_lib/Mechanical/Translational Elements/Translational Damper  Tag=Factory Generic  D=362 N/(m/s)  v_specify=off  v_priority=High  v=0 m/s  v_nominal_specify=off  v_nominal_unit=m/s  v_nominal_value=1  f_specify=off  f_priority=High  f=0 N  f_nominal_specify=off  f_nominal_unit=N  f_nominal_value=1
  Spool Mass : fl_lib/Mechanical/Translational Elements/Mass  Tag=Factory Generic  mass=0.124 kg  num_ports=foundation.enum.numPorts2.one  v_specify=on  v_priority=High  v=0 m/s  v_nominal_specify=off  v_nominal_unit=m/s  v_nominal_value=1  f_specify=off  f_priority=High  f=0 N  f_nominal_specify=off  f_nominal_unit=N  f_nominal_value=1
  Spool Side A : Subsystem
  Spool Side B : Subsystem
  A_S : PMIOPort  Side=Left
  Flapper : PMIOPort  Port=2  Side=Left
  B_S : PMIOPort  Port=3  Side=Left
  A : PMIOPort  Port=4  Side=Right
  P : PMIOPort  Port=5  Side=Right
  B : PMIOPort  Port=6  Side=Right
  T : PMIOPort  Port=7  Side=Right
  connections:
  A/RConn1 -- Orifice AT/LConn2 -- Orifice PA/RConn1
  P/RConn1 -- Orifice PB/LConn2 -- Orifice PA/LConn2
  Orifice BT/LConn2 -- Orifice PB/RConn1 -- B/RConn1
  T/RConn1 -- Orifice AT/RConn1 -- Orifice BT/RConn1
  MTRef Spool A/LConn1 -- Spool Damper/RConn1 -- Spool Side A/LConn1
  A_S/RConn1 -- Spool Side A/LConn2
  Orifice PA/LConn1 -- Orifice PB/LConn1 -- Orifice BT/LConn1 -- Orifice AT/LConn1 -- Spool Side B/RConn1 -- Spool Side A/RConn1 -- Spool Damper/LConn1 -- Spool Mass/LConn1 -- Flapper/RConn1
  Spool Side B/LConn1 -- MTRef Spool B/LConn1
  Spool Side B/LConn2 -- B_S/RConn1

== system pha_0_5_servovalve/Servovalve/Nozzle A ==
  Nozzle A : SimscapeFluids_lib/Isothermal Liquid/Valves & Orifices/Orifices/Orifice (IL)  Tag=Factory Generic  orifice_type=foundation.enum.constant_variable.variable  constant_orifice_spec=fluids.isothermal_liquid.valves_orifices.orifices.enum.constant_orifice_spec.area  variable_orifice_spec=1  orifice_area_constant=1e-3 m^2  p_diff_TLU_constant=[-4, -3, -2, -1, -.5, 0, .5, 1, 2, 3, 4] MPa  vol_flow_TLU_constant=[-2.44, -2.12, -1.68, -1.22, -.84, 0, .85, 1.21, 1.7, 2.09, 2.41] .* 1e-3 m^3/s  S_min=-2.9981e-07 m^2/mm  del_S=5.9981e-07 m^2/mm  open_orientation=1  area_max=3.14 mm^2  area_leak=1e-9 m^2  S_TLU="[  -0.002 0 0.005 0.015 ] - 0.001*(0.3) m"  orifice_area_TLU="[  1e-12 4e-12 1e-05 1.02e-05 ] m^2"  area=inf m^2  Cd=0.7  Re_c=150  smoothing_factor=0  pressure_recovery=false  S_vol_flow_TLU="[  -0.002 0 0.005 0.015 ] - 0.001*(0.3) m"  p_diff_TLU="[  -5e+06 -2e+06 2e+06 5e+06 ] Pa"  vol_flow_TLU="[  -1e-12 -6e-14 6e+12 1e+11 ; -8e-08 -4e-08 4e+06 8e+06 ; -0.0025 -0.00103 0.001 0.0024 ; -0.00258 -0.001032 0.00106 0.00247 ; ] m^3/s"  enable_faults=simscape.enum.onoff.off  fault_action=fluids.enum.FaultOpening.Closed  external_fault=fluids.enum.FaultExternalTrigger.Off  temporal_fault=simscape.enum.onoff.off  fault_time=5 s  report_fault=simscape.enum.assert.action.none
      settings: InternalSimscapePortConfiguration="{\"Bottom\":[],\"Left\":[{\"id\":\"A\",\"label\":\"A\",\"type\":\"foundation.isothermal_liquid.isothermal_liquid\"},{\"id\":\"S\",\"label\":\"S\",\"type\":\"input\"}],\"Right\":[{\"id\":\"B\",\"label\":\"B\",\"type\":\"foundation.isothermal_liquid.isothermal_liquid\"}],\"Top\":[]}"
  S : PMIOPort  Side=Left
  A : PMIOPort  Port=2  Side=Left
  B : PMIOPort  Port=3  Side=Right
  connections:
  Nozzle A/LConn1 -- A/RConn1
  Nozzle A/LConn2 -- S/RConn1
  B/RConn1 -- Nozzle A/RConn1

== system pha_0_5_servovalve/Servovalve/Nozzle B ==
  Nozzle B : SimscapeFluids_lib/Isothermal Liquid/Valves & Orifices/Orifices/Orifice (IL)  Tag=Factory Generic  orifice_type=foundation.enum.constant_variable.variable  constant_orifice_spec=fluids.isothermal_liquid.valves_orifices.orifices.enum.constant_orifice_spec.area  variable_orifice_spec=1  orifice_area_constant=1e-3 m^2  p_diff_TLU_constant=[-4, -3, -2, -1, -.5, 0, .5, 1, 2, 3, 4] MPa  vol_flow_TLU_constant=[-2.44, -2.12, -1.68, -1.22, -.84, 0, .85, 1.21, 1.7, 2.09, 2.41] .* 1e-3 m^3/s  S_min=2.9981e-07 m^2/mm  del_S=5.9981e-07 m^2/mm  open_orientation=-1  area_max=3.14 mm^2  area_leak=1e-9 m^2  S_TLU="-([  -0.002 0 0.005 0.015 ]) + 0.001*(0.3) m"  orifice_area_TLU="[  1e-12 4e-12 1e-05 1.02e-05 ] m^2"  area=inf m^2  Cd=0.7  Re_c=150  smoothing_factor=0  pressure_recovery=false  S_vol_flow_TLU="-([  -0.002 0 0.005 0.015 ]) + 0.001*(0.3) m"  p_diff_TLU="[  -5e+06 -2e+06 2e+06 5e+06 ] Pa"  vol_flow_TLU="[  -1e-12 -6e-14 6e+12 1e+11 ; -8e-08 -4e-08 4e+06 8e+06 ; -0.0025 -0.00103 0.001 0.0024 ; -0.00258 -0.001032 0.00106 0.00247 ; ] m^3/s"  enable_faults=simscape.enum.onoff.off  fault_action=fluids.enum.FaultOpening.Closed  external_fault=fluids.enum.FaultExternalTrigger.Off  temporal_fault=simscape.enum.onoff.off  fault_time=5 s  report_fault=simscape.enum.assert.action.none
      settings: InternalSimscapePortConfiguration="{\"Bottom\":[],\"Left\":[{\"id\":\"A\",\"label\":\"A\",\"type\":\"foundation.isothermal_liquid.isothermal_liquid\"},{\"id\":\"S\",\"label\":\"S\",\"type\":\"input\"}],\"Right\":[{\"id\":\"B\",\"label\":\"B\",\"type\":\"foundation.isothermal_liquid.isothermal_liquid\"}],\"Top\":[]}"
  S : PMIOPort  Side=Left
  A : PMIOPort  Port=2  Side=Left
  B : PMIOPort  Port=3  Side=Right
  connections:
  A/RConn1 -- Nozzle B/LConn1
  S/RConn1 -- Nozzle B/LConn2
  B/RConn1 -- Nozzle B/RConn1

== system pha_0_5_servovalve/Servovalve1/Fixed Orifice A ==
  Fixed Orifice A : SimscapeFluids_lib/Isothermal Liquid/Valves & Orifices/Orifices/Orifice (IL)  Tag=Factory Generic  orifice_type=1  constant_orifice_spec=fluids.isothermal_liquid.valves_orifices.orifices.enum.constant_orifice_spec.area  variable_orifice_spec=fluids.isothermal_liquid.valves_orifices.orifices.enum.orifice_spec.linear  orifice_area_constant=2 mm^2  p_diff_TLU_constant=[-4, -3, -2, -1, -.5, 0, .5, 1, 2, 3, 4] MPa  vol_flow_TLU_constant=[-2.44, -2.12, -1.68, -1.22, -.84, 0, .85, 1.21, 1.7, 2.09, 2.41] .* 1e-3 m^3/s  S_min=0 m  del_S=5e-3 m  open_orientation=fluids.isothermal_liquid.valves_orifices.orifices.enum.orifice_orientation.positive  area_max=1e-4 m^2  area_leak=1e-10 m^2  S_TLU=[0, .002, .004, .007, .017] m  orifice_area_TLU=[1e-09, 2.0352e-07, 4.0736e-05, .00011438, .00034356] m^2  area=inf mm^2  Cd=0.7  Re_c=150  smoothing_factor=0.01  pressure_recovery=false  S_vol_flow_TLU=[0, .002, .004, .007, .017] m  p_diff_TLU=[.3, .5, .7] MPa  vol_flow_TLU=1e-3 * [1.7e-05, 2e-05, 2.6e-05; .0035, .0045, .0053; .7, .9, 1.06; 1.96, 2.5, 3; 6, 7.7, 9.13] m^3/s  enable_faults=simscape.enum.onoff.off  fault_action=fluids.enum.FaultOpening.Closed  external_fault=fluids.enum.FaultExternalTrigger.Off  temporal_fault=simscape.enum.onoff.off  fault_time=5 s  report_fault=simscape.enum.assert.action.none
      settings: InternalSimscapePortConfiguration="{\"Bottom\":[],\"Left\":[{\"id\":\"A\",\"label\":\"A\",\"type\":\"foundation.isothermal_liquid.isothermal_liquid\"}],\"Right\":[{\"id\":\"B\",\"label\":\"B\",\"type\":\"foundation.isothermal_liquid.isothermal_liquid\"}],\"Top\":[]}"
  B : PMIOPort  Side=Right
  A : PMIOPort  Port=2  Side=Left
  connections:
  A/RConn1 -- Fixed Orifice A/LConn1
  B/RConn1 -- Fixed Orifice A/RConn1

== system pha_0_5_servovalve/Servovalve1/Fixed Orifice B ==
  Fixed Orifice B : SimscapeFluids_lib/Isothermal Liquid/Valves & Orifices/Orifices/Orifice (IL)  Tag=Factory Generic  orifice_type=1  constant_orifice_spec=fluids.isothermal_liquid.valves_orifices.orifices.enum.constant_orifice_spec.area  variable_orifice_spec=fluids.isothermal_liquid.valves_orifices.orifices.enum.orifice_spec.linear  orifice_area_constant=2 mm^2  p_diff_TLU_constant=[-4, -3, -2, -1, -.5, 0, .5, 1, 2, 3, 4] MPa  vol_flow_TLU_constant=[-2.44, -2.12, -1.68, -1.22, -.84, 0, .85, 1.21, 1.7, 2.09, 2.41] .* 1e-3 m^3/s  S_min=0 m  del_S=5e-3 m  open_orientation=fluids.isothermal_liquid.valves_orifices.orifices.enum.orifice_orientation.positive  area_max=1e-4 m^2  area_leak=1e-10 m^2  S_TLU=[0, .002, .004, .007, .017] m  orifice_area_TLU=[1e-09, 2.0352e-07, 4.0736e-05, .00011438, .00034356] m^2  area=inf mm^2  Cd=0.7  Re_c=150  smoothing_factor=0.01  pressure_recovery=false  S_vol_flow_TLU=[0, .002, .004, .007, .017] m  p_diff_TLU=[.3, .5, .7] MPa  vol_flow_TLU=1e-3 * [1.7e-05, 2e-05, 2.6e-05; .0035, .0045, .0053; .7, .9, 1.06; 1.96, 2.5, 3; 6, 7.7, 9.13] m^3/s  enable_faults=simscape.enum.onoff.off  fault_action=fluids.enum.FaultOpening.Closed  external_fault=fluids.enum.FaultExternalTrigger.Off  temporal_fault=simscape.enum.onoff.off  fault_time=5 s  report_fault=simscape.enum.assert.action.none
      settings: InternalSimscapePortConfiguration="{\"Bottom\":[],\"Left\":[{\"id\":\"A\",\"label\":\"A\",\"type\":\"foundation.isothermal_liquid.isothermal_liquid\"}],\"Right\":[{\"id\":\"B\",\"label\":\"B\",\"type\":\"foundation.isothermal_liquid.isothermal_liquid\"}],\"Top\":[]}"
  B : PMIOPort  Side=Right
  A : PMIOPort  Port=2  Side=Left
  connections:
  A/RConn1 -- Fixed Orifice B/LConn1
  B/RConn1 -- Fixed Orifice B/RConn1

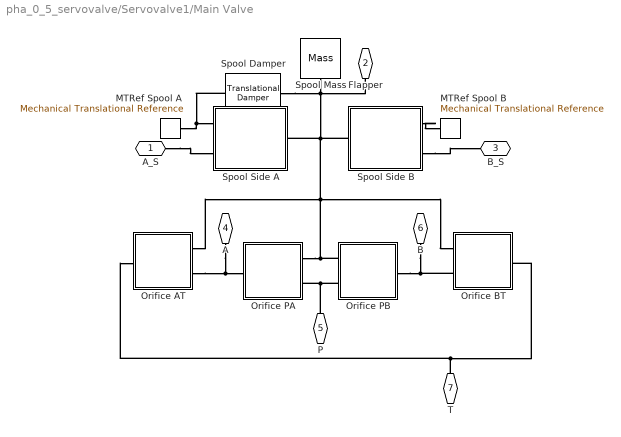
== system pha_0_5_servovalve/Servovalve1/Main Valve ==
  MTRef Spool A : fl_lib/Mechanical/Translational Elements/Mechanical Translational Reference  Tag=Factory Generic
  MTRef Spool B : fl_lib/Mechanical/Translational Elements/Mechanical Translational Reference  Tag=Factory Generic
  Orifice AT : Subsystem  Tag=PublishSubsystem
  Orifice BT : Subsystem
  Orifice PA : Subsystem
  Orifice PB : Subsystem
  Spool Damper : fl_lib/Mechanical/Translational Elements/Translational Damper  Tag=Factory Generic  D=362 N/(m/s)  v_specify=off  v_priority=High  v=0 m/s  v_nominal_specify=off  v_nominal_unit=m/s  v_nominal_value=1  f_specify=off  f_priority=High  f=0 N  f_nominal_specify=off  f_nominal_unit=N  f_nominal_value=1
  Spool Mass : fl_lib/Mechanical/Translational Elements/Mass  Tag=Factory Generic  mass=0.124 kg  num_ports=foundation.enum.numPorts2.one  v_specify=on  v_priority=High  v=0 m/s  v_nominal_specify=off  v_nominal_unit=m/s  v_nominal_value=1  f_specify=off  f_priority=High  f=0 N  f_nominal_specify=off  f_nominal_unit=N  f_nominal_value=1
  Spool Side A : Subsystem
  Spool Side B : Subsystem
  A_S : PMIOPort  Side=Left
  Flapper : PMIOPort  Port=2  Side=Left
  B_S : PMIOPort  Port=3  Side=Left
  A : PMIOPort  Port=4  Side=Right
  P : PMIOPort  Port=5  Side=Right
  B : PMIOPort  Port=6  Side=Right
  T : PMIOPort  Port=7  Side=Right
  connections:
  A/RConn1 -- Orifice AT/LConn2 -- Orifice PA/RConn1
  P/RConn1 -- Orifice PB/LConn2 -- Orifice PA/LConn2
  Orifice BT/LConn2 -- Orifice PB/RConn1 -- B/RConn1
  T/RConn1 -- Orifice AT/RConn1 -- Orifice BT/RConn1
  MTRef Spool A/LConn1 -- Spool Damper/RConn1 -- Spool Side A/LConn1
  A_S/RConn1 -- Spool Side A/LConn2
  Orifice PA/LConn1 -- Orifice PB/LConn1 -- Orifice BT/LConn1 -- Orifice AT/LConn1 -- Spool Side B/RConn1 -- Spool Side A/RConn1 -- Spool Damper/LConn1 -- Spool Mass/LConn1 -- Flapper/RConn1
  Spool Side B/LConn1 -- MTRef Spool B/LConn1
  Spool Side B/LConn2 -- B_S/RConn1

== system pha_0_5_servovalve/Servovalve1/Nozzle A ==
  Nozzle A : SimscapeFluids_lib/Isothermal Liquid/Valves & Orifices/Orifices/Orifice (IL)  Tag=Factory Generic  orifice_type=foundation.enum.constant_variable.variable  constant_orifice_spec=fluids.isothermal_liquid.valves_orifices.orifices.enum.constant_orifice_spec.area  variable_orifice_spec=1  orifice_area_constant=1e-3 m^2  p_diff_TLU_constant=[-4, -3, -2, -1, -.5, 0, .5, 1, 2, 3, 4] MPa  vol_flow_TLU_constant=[-2.44, -2.12, -1.68, -1.22, -.84, 0, .85, 1.21, 1.7, 2.09, 2.41] .* 1e-3 m^3/s  S_min=-2.9981e-07 m^2/mm  del_S=5.9981e-07 m^2/mm  open_orientation=1  area_max=3.14 mm^2  area_leak=1e-9 m^2  S_TLU="[  -0.002 0 0.005 0.015 ] - 0.001*(0.3) m"  orifice_area_TLU="[  1e-12 4e-12 1e-05 1.02e-05 ] m^2"  area=inf m^2  Cd=0.7  Re_c=150  smoothing_factor=0  pressure_recovery=false  S_vol_flow_TLU="[  -0.002 0 0.005 0.015 ] - 0.001*(0.3) m"  p_diff_TLU="[  -5e+06 -2e+06 2e+06 5e+06 ] Pa"  vol_flow_TLU="[  -1e-12 -6e-14 6e+12 1e+11 ; -8e-08 -4e-08 4e+06 8e+06 ; -0.0025 -0.00103 0.001 0.0024 ; -0.00258 -0.001032 0.00106 0.00247 ; ] m^3/s"  enable_faults=simscape.enum.onoff.off  fault_action=fluids.enum.FaultOpening.Closed  external_fault=fluids.enum.FaultExternalTrigger.Off  temporal_fault=simscape.enum.onoff.off  fault_time=5 s  report_fault=simscape.enum.assert.action.none
      settings: InternalSimscapePortConfiguration="{\"Bottom\":[],\"Left\":[{\"id\":\"A\",\"label\":\"A\",\"type\":\"foundation.isothermal_liquid.isothermal_liquid\"},{\"id\":\"S\",\"label\":\"S\",\"type\":\"input\"}],\"Right\":[{\"id\":\"B\",\"label\":\"B\",\"type\":\"foundation.isothermal_liquid.isothermal_liquid\"}],\"Top\":[]}"
  S : PMIOPort  Side=Left
  A : PMIOPort  Port=2  Side=Left
  B : PMIOPort  Port=3  Side=Right
  connections:
  Nozzle A/LConn1 -- A/RConn1
  Nozzle A/LConn2 -- S/RConn1
  B/RConn1 -- Nozzle A/RConn1
